simulink library "UR3_Lib"  (R2017a)
settings: Solver=VariableStepAuto  StartTime=0.0  StopTime=10.0  RelTol=1e-3
settings Model: Creator=dscat  LastModifiedBy=dscat

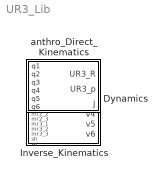
== system UR3_Lib ==
  Dynamics : MATLAB Function  TreatAsAtomicUnit=on
  Inverse_Kinematics : MATLAB Function  TreatAsAtomicUnit=on
  anthro_Direct_Kinematics : MATLAB Function  TreatAsAtomicUnit=on

== matlab function UR3_Lib/Inverse_Kinematics ==
  data: el input; v1 output; mp1 input; mp2 input; mp3 input; mr1_1 input; mr1_2 input; mr1_3 input; mr2_1 input; mr2_2 input; mr2_3 input; mr3_1 input; mr3_2 input; mr3_3 input; sh input; wr input; v2 output; v3 output; v4 output; v5 output; v6 output
function [v1,v2,v3,v4,v5,v6] = Inverse_Kinematics(el,mp1,mp2,mp3,mr1_1,mr1_2,mr1_3,mr2_1,mr2_2,mr2_3,mr3_1,mr3_2,mr3_3,sh,wr)
%#codegen

%    This function was generated by the Symbolic Math Toolbox version 7.2.
%    02-Jun-2018 14:50:33

t6 = mr1_3.*(4.1e1./5.0e2);
t2 = mp1-t6;
t9 = mr2_3.*(4.1e1./5.0e2);
t3 = mp2-t9;
t4 = pi.*(1.0./2.0);
t5 = mp2.*1i;
t7 = mr2_3.*-8.2e-2i;
t8 = t2.^2;
t10 = t3.^2;
t11 = t8+t10;
t12 = 1.0./sqrt(t11);
t13 = t12.*(1.1e1./1.0e2);
t14 = acos(t13);
t15 = sh.*t14;
v1 = t4+t15+angle(mp1-mr1_3.*(4.1e1./5.0e2)+t5+t7);
if nargout > 1
    t16 = mp1+t5-t6+t7;
    t17 = angle(t16);
    t18 = t4+t15+t17;
    t19 = cos(t18);
    t20 = sin(t18);
    t21 = t19.^2;
    t22 = t20.^2;
    t23 = t21+t22;
    t24 = 1.0./t23;
    t25 = mp1.*t20.*(5.0e2./4.1e1);
    t31 = mp2.*t19.*(5.0e2./4.1e1);
    t26 = t25-t31-5.5e1./4.1e1;
    t27 = acos(t26);
    t28 = t27.*wr;
    t29 = sin(t28);
    t30 = 1.0./t29;
    t32 = cos(t28);
    t33 = mr1_2.*t20;
    t38 = mr2_2.*t19;
    t34 = t33-t38;
    t35 = mr1_1.*t20;
    t37 = mr2_1.*t19;
    t36 = t35-t37;
    t44 = t30.*t34;
    t39 = real(-t44);
    t42 = t30.*t36;
    t40 = imag(-t42);
    t41 = t39-t40;
    t116 = t30.*(t33-t38).*-1i;
    t43 = -t116;
    t45 = -t42+t43;
    t46 = abs(t45);
    t47 = t32.^2;
    t48 = real(-t42);
    t49 = imag(-t44);
    t50 = t48+t49;
    t51 = 1.0./t46.^2;
    t52 = t29.^2;
    t53 = t50.^2;
    t54 = t41.^2;
    t55 = 1.0./t46;
    t56 = t47.*t51.*t53;
    t57 = t51.*t52.*t53;
    t58 = t47.*t51.*t54;
    t59 = t51.*t52.*t54;
    t60 = t56+t57+t58+t59;
    t61 = 1.0./t60;
    t63 = t47.*t50.*t55.*8.3e1;
    t64 = t29.*t41.*t55.*1.1e2;
    t65 = t50.*t52.*t55.*8.3e1;
    t66 = t63-t64+t65;
    t67 = t29.*t50.*t55.*1.1e2;
    t68 = t47+t52;
    t69 = 1.0./t68;
    t70 = t32.*5.5e1;
    t71 = t47.*4.1e1;
    t72 = t52.*4.1e1;
    t73 = t70+t71+t72;
    t81 = mr1_1.*t19.*t24;
    t82 = mr2_1.*t20.*t24;
    t83 = t81+t82;
    t84 = mp1.*t19.*t24;
    t85 = mp2.*t20.*t24;
    t86 = mr1_3.*t19.*t24;
    t87 = mr2_3.*t20.*t24;
    t88 = t86+t87;
    t89 = t69.*t73.*t88.*(1.0./5.0e2);
    t90 = mr1_2.*t19.*t24;
    t91 = mr2_2.*t20.*t24;
    t92 = t90+t91;
    t93 = t61.*t66.*t92.*(1.0./1.0e3);
    t62 = t84+t85-t89-t93+t61.*t83.*(t67+(t41.*t52.*8.3e1)./abs(t43-t30.*t36)+(t41.*t47.*8.3e1)./abs(t30.*t34.*1i-t30.*t36)).*(1.0./1.0e3);
    t75 = mr3_2.*t61.*t66.*(1.0./1.0e3);
    t76 = t41.*t47.*t55.*8.3e1;
    t77 = t41.*t52.*t55.*8.3e1;
    t78 = t67+t76+t77;
    t79 = mr3_1.*t61.*t78.*(1.0./1.0e3);
    t80 = mr3_3.*t69.*t73.*(1.0./5.0e2);
    t74 = mp3-t75+t79-t80;
    t97 = t61.*t78.*t83.*(1.0./1.0e3);
    t94 = t84+t85-t89-t93+t97;
    t95 = t74.^2;
    t98 = t94.^2;
    t100 = t98.*9.620564919572077;
    t101 = t95.*9.620564919572077;
    t96 = t100+t101-1.009245362887709;
    t99 = t95.*(1.25e2./6.1e1);
    t102 = t96.^2;
    t103 = -t102+1.0;
    t104 = sqrt(t103);
    t105 = t95+t98;
    t106 = 1.0./t105;
    t107 = el.*t104.*1i;
    t108 = t100+t101+t107-1.009245362887709;
    t109 = angle(t108);
    t110 = t98.*(1.25e2./6.1e1);
    t111 = t99+t110+2.903073770491803e-2;
    t112 = t94.*t111;
    t113 = el.*t74.*t104.*(2.13e2./1.0e3);
    t114 = t112+t113;
    t115 = t106.*t114.*1i;
    v2 = -angle(t115+t106.*(t74.*(t99+t62.^2.*(1.25e2./6.1e1)+2.903073770491803e-2)-el.*t94.*t104.*(2.13e2./1.0e3)));
end
if nargout > 2
    v3 = t109;
end
if nargout > 3
    v4 = -t109+angle(t115+t106.*(t74.*t111-el.*t94.*t104.*(2.13e2./1.0e3)))+angle(-mr3_1.*t41.*t55+mr3_2.*t50.*t55+mr1_1.*t19.*t41.*t55.*1i-mr1_2.*t19.*t50.*t55.*1i+mr2_1.*t20.*t41.*t55.*1i-mr2_2.*t20.*t50.*t55.*1i);
end
if nargout > 4
    v5 = t28;
end
if nargout > 5
    v6 = angle(t116+t30.*(t35-t37));
end

== matlab function UR3_Lib/anthro_Direct_Kinematics ==
  data: q1 input; UR3_R output; q2 input; q3 input; q4 input; q5 input; q6 input; UR3_p output; J output
function [UR3_R,UR3_p,J] = anthro_Direct_Kinematics(q1,q2,q3,q4,q5,q6)
%#codegen

%    This function was generated by the Symbolic Math Toolbox version 7.2.
%    02-Jun-2018 14:45:26

t2 = cos(q1);
t3 = cos(q2);
t4 = cos(q5);
t5 = cos(q3);
t6 = sin(q4);
t7 = cos(q4);
t8 = sin(q2);
t9 = sin(q3);
t10 = sin(q6);
t11 = sin(q1);
t12 = sin(q5);
t13 = t11.*t12;
t14 = t2.*t3.*t4.*t6.*t9;
t15 = t2.*t4.*t5.*t6.*t8;
t16 = t2.*t4.*t7.*t8.*t9;
t17 = t13+t14+t15+t16-t2.*t3.*t4.*t5.*t7;
t18 = q2+q3+q4;
t19 = sin(t18);
t20 = cos(q6);
t21 = t3.*t4.*t6.*t9.*t11;
t22 = t4.*t5.*t6.*t8.*t11;
t23 = t4.*t7.*t8.*t9.*t11;
t24 = t21+t22+t23-t2.*t12-t3.*t4.*t5.*t7.*t11;
t25 = q2+q3+q4+q6;
t26 = q2+q3+q4-q6;
t27 = q2+q3+q4+q5;
t28 = cos(t27);
t29 = q2+q3+q4-q5;
t30 = cos(t29);
t31 = t6.*t8.*t9.*t11.*(8.3e1./1.0e3);
t32 = t3.*t5.*t7.*t11.*t12.*(4.1e1./5.0e2);
t33 = cos(t18);
t34 = t33.*(8.3e1./1.0e3);
t35 = q2+q3;
t36 = cos(t35);
t37 = t36.*(2.13e2./1.0e3);
t38 = t3.*(6.1e1./2.5e2);
t39 = t30.*(4.1e1./1.0e3);
t41 = t28.*(4.1e1./1.0e3);
t40 = t34+t37+t38+t39-t41;
t42 = t2.*t4.*(4.1e1./5.0e2);
t43 = t3.*t5.*t6.*t11.*(8.3e1./1.0e3);
t44 = t3.*t7.*t9.*t11.*(8.3e1./1.0e3);
t45 = t5.*t7.*t8.*t11.*(8.3e1./1.0e3);
t46 = t3.*t6.*t9.*t11.*t12.*(4.1e1./5.0e2);
t47 = t5.*t6.*t8.*t11.*t12.*(4.1e1./5.0e2);
t48 = t7.*t8.*t9.*t11.*t12.*(4.1e1./5.0e2);
t49 = t34+t39-t41;
t50 = t3.*t5.*t7.*t11.*t12;
t51 = t30.*(1.0./2.0);
t52 = t11.*(1.1e1./1.0e2);
t53 = t4.*t11.*(4.1e1./5.0e2);
t54 = t2.*t6.*t8.*t9.*(8.3e1./1.0e3);
t55 = t2.*t3.*t5.*t7.*t12.*(4.1e1./5.0e2);
t60 = t2.*t3.*t5.*t6.*(8.3e1./1.0e3);
t61 = t2.*t3.*t7.*t9.*(8.3e1./1.0e3);
t62 = t2.*t5.*t7.*t8.*(8.3e1./1.0e3);
t63 = t2.*t3.*t6.*t9.*t12.*(4.1e1./5.0e2);
t64 = t2.*t5.*t6.*t8.*t12.*(4.1e1./5.0e2);
t65 = t2.*t7.*t8.*t9.*t12.*(4.1e1./5.0e2);
t75 = t2.*t8.*(6.1e1./2.5e2);
t76 = t2.*t3.*t9.*(2.13e2./1.0e3);
t77 = t2.*t5.*t8.*(2.13e2./1.0e3);
t56 = t52+t53+t54+t55-t60-t61-t62-t63-t64-t65-t75-t76-t77;
t57 = t34+t37+t39-t41;
t58 = q1+q2+q3+q4;
t59 = -q1+q2+q3+q4;
t66 = t4.*t11;
t67 = t2.*t3.*t5.*t7.*t12;
UR3_R = reshape([t17.*t20+t2.*t10.*t19,t20.*t24+t10.*t11.*t19,sin(t25).*(-1.0./2.0)+sin(t26).*(1.0./2.0)-t4.*t19.*t20,-t10.*t17+t2.*t19.*t20,-t10.*t24+t11.*t19.*t20,cos(t25).*(-1.0./2.0)-cos(t26).*(1.0./2.0)+t4.*t10.*t19,t66+t67-t2.*t3.*t6.*t9.*t12-t2.*t5.*t6.*t8.*t12-t2.*t7.*t8.*t9.*t12,t50-t2.*t4-t3.*t6.*t9.*t11.*t12-t5.*t6.*t8.*t11.*t12-t7.*t8.*t9.*t11.*t12,t28.*(-1.0./2.0)+t51],[3,3]);
if nargout > 1
    UR3_p = [t56;t2.*(-1.1e1./1.0e2)+t31+t32-t2.*t4.*(4.1e1./5.0e2)-t8.*t11.*(6.1e1./2.5e2)-t3.*t9.*t11.*(2.13e2./1.0e3)-t5.*t8.*t11.*(2.13e2./1.0e3)-t3.*t5.*t6.*t11.*(8.3e1./1.0e3)-t3.*t7.*t9.*t11.*(8.3e1./1.0e3)-t5.*t7.*t8.*t11.*(8.3e1./1.0e3)-t3.*t6.*t9.*t11.*t12.*(4.1e1./5.0e2)-t5.*t6.*t8.*t11.*t12.*(4.1e1./5.0e2)-t7.*t8.*t9.*t11.*t12.*(4.1e1./5.0e2);t40];
end
if nargout > 2
    t68 = t28.*(1.0./2.0);
    t69 = t51-t68;
    t70 = t2.*(1.1e1./1.0e2);
    t71 = t8.*t11.*(6.1e1./2.5e2);
    t72 = t3.*t9.*t11.*(2.13e2./1.0e3);
    t73 = t5.*t8.*t11.*(2.13e2./1.0e3);
    t74 = -t31-t32+t42+t43+t44+t45+t46+t47+t48+t70+t71+t72+t73;
    t78 = sin(t35);
    t79 = t78.*2.13e2;
    t80 = t8.*2.44e2;
    t81 = t79+t80;
    t82 = cos(t58);
    t83 = t82.*(1.0./2.0);
    t84 = cos(t59);
    t104 = t84.*(1.0./2.0);
    t85 = t83-t104;
    t86 = -t53-t54-t55+t60+t61+t62+t63+t64+t65;
    t87 = sin(t58);
    t88 = t87.*(1.0./2.0);
    t89 = sin(t59);
    t90 = t89.*(1.0./2.0);
    t91 = t88+t90;
    t92 = -t31-t32+t42+t43+t44+t45+t46+t47+t48;
    t93 = -t53-t55+t63+t64+t65;
    t94 = t2.*t4;
    t95 = t3.*t6.*t9.*t11.*t12;
    t96 = t5.*t6.*t8.*t11.*t12;
    t97 = t7.*t8.*t9.*t11.*t12;
    t98 = -t50+t94+t95+t96+t97;
    t99 = t2.*t3.*t6.*t9.*t12;
    t100 = t2.*t5.*t6.*t8.*t12;
    t101 = t2.*t7.*t8.*t9.*t12;
    t102 = -t66-t67+t99+t100+t101;
    t103 = -t32+t42+t46+t47+t48;
    J = reshape([t74,t56,0.0,0.0,0.0,1.0,-t2.*t40,-t11.*t40,-t11.*t74-t2.*(-t52-t53-t54-t55+t60+t61+t62+t63+t64+t65+t75+t76+t77),t11,-t2,0.0,-t2.*t57,-t11.*t57,-t2.*(-t52-t53-t54-t55+t60+t61+t62+t63+t64+t65+t76+t77)-t11.*(-t31-t32+t42+t43+t44+t45+t46+t47+t48+t70+t72+t73),t11,-t2,0.0,-t2.*t49,-t11.*t49,-t11.*(-t31-t32+t42+t43+t44+t45+t46+t47+t48+t70+t71+t72+t73-t11.*t81.*(1.0./1.0e3))-t2.*(-t52-t53-t54-t55+t60+t61+t62+t63+t64+t65+t75+t76+t77-t2.*t81.*(1.0./1.0e3)),t11,-t2,0.0,t33.*t92+t49.*t85,-t33.*t86+t49.*t91,t85.*t86+t91.*t92,-t88-t90,t85,t33,t69.*t103-t98.*(t39-t41),-t69.*t93+t102.*(t39-t41),-t93.*t98+t102.*t103,t66+t67-t99-t100-t101,t50-t94-t95-t96-t97,t69],[6,6]);
end

== matlab function UR3_Lib/Dynamics ==
  data: dq1 input; G output; dq2 input; dq3 input; dq4 input; dq5 input; dq6 input; q2 input; q3 input; q4 input; q5 input; q6 input; C_dq output; B output
function [G,C_dq,B] = Dynamics(dq1,dq2,dq3,dq4,dq5,dq6,q2,q3,q4,q5,q6)
%#codegen

%    This function was generated by the Symbolic Math Toolbox version 7.2.
%    02-Jun-2018 15:14:17

t2 = cos(q2);
t3 = sin(q3);
t4 = cos(q3);
t5 = sin(q2);
t6 = sin(q4);
t7 = cos(q5);
t8 = cos(q4);
t9 = t2.*t3.*(9.81e2./1.0e2);
t10 = t4.*t5.*(9.81e2./1.0e2);
t11 = t9+t10;
t12 = t8.*t11;
t13 = t2.*t4.*(9.81e2./1.0e2);
t17 = t3.*t5.*(9.81e2./1.0e2);
t14 = t13-t17;
t15 = t6.*t14;
t16 = t12+t15;
t18 = cos(q6);
t19 = sin(q6);
t20 = t6.*t11;
t22 = t8.*t14;
t21 = t20-t22;
t23 = sin(q5);
t24 = t7.*t16.*3.3852e-1;
t25 = t19.*t21.*1.6113e-1;
t31 = t7.*t16.*t18.*1.6113e-1;
t26 = t25-t31;
t27 = t18.*t21.*1.6113e-1;
t28 = t7.*t16.*t19.*1.6113e-1;
t37 = t27+t28;
t29 = t19.*t37;
t38 = t18.*t26;
t30 = t24+t29-t38;
t32 = t18.*t21.*1.06974207e-2;
t33 = t7.*t16.*t19.*1.06974207e-2;
t34 = t32+t33;
t35 = t19.*t21.*1.06974207e-2;
t40 = t7.*t16.*t18.*1.06974207e-2;
t36 = t35-t40;
t39 = t7.*t16.*4.5395532e-3;
t41 = t23.^2;
t42 = t16.*t41.*5.49615e-2;
t43 = t8.*t11.*3.7397712e-2;
t44 = t6.*t14.*3.7397712e-2;
t45 = t7.*t16.*3.00842724e-2;
t46 = t16.*t23.*4.34580624e-2;
t47 = t18.*t34;
t48 = t19.*t36;
t49 = t6.*t11.*4.5395532e-3;
t63 = t8.*t14.*4.5395532e-3;
t50 = t46+t47+t48+t49-t63;
t51 = t7.*t50;
t52 = t18.*t37.*(1.1e1./1.0e2);
t53 = t6.*t11.*7.4634912e-2;
t54 = t19.*t26.*(1.1e1./1.0e2);
t55 = t2.*t4.*1.02069867636e-1;
t56 = t19.*(t27+t28);
t57 = t24-t38+t56;
t58 = t7.*t57.*(1.1e1./1.0e2);
t59 = t19.*(t32+t33);
t72 = t18.*t36;
t60 = t39+t42+t43+t44+t58+t59-t72;
t61 = t19.*(t27+t28).*(8.3e1./1.0e3);
t76 = t18.*t26.*(8.3e1./1.0e3);
t62 = t45+t61-t76;
t77 = t23.*t62;
t78 = t8.*t14.*7.4634912e-2;
t64 = t51+t52+t53+t54-t77-t78;
t65 = t4.^2;
t66 = t65.*(2.13e2./1.0e3);
t67 = t3.^2;
t68 = t67.*(2.13e2./1.0e3);
t69 = t66+t68-1.1812e-1;
t70 = t23.*t57;
t107 = t7.*t16.*t23.*4.9965e-1;
t71 = t70-t107;
t73 = t8.*t60;
t74 = t2.*t3.*1.02069867636e-1;
t75 = t4.*t5.*1.02069867636e-1;
t79 = t6.*t64;
t80 = t73+t74+t75+t79;
t81 = t7.*t57;
t82 = t16.*t41.*4.9965e-1;
t83 = t8.*t11.*3.2195e-1;
t84 = t6.*t14.*3.2195e-1;
t85 = t81+t82+t83+t84;
t86 = t18.*t37;
t87 = t6.*t11.*6.6047e-1;
t88 = t19.*t26;
t98 = t8.*t14.*6.6047e-1;
t89 = t86+t87+t88-t98;
t90 = t2.^2;
t91 = t90.*(6.1e1./2.5e2);
t92 = t5.^2;
t93 = t92.*(6.1e1./2.5e2);
t94 = t91+t93-1.6e1./1.25e2;
t95 = t2.*t3.*1.03205124e1;
t96 = t4.*t5.*1.03205124e1;
t97 = t8.*t85;
t99 = t6.*t89;
t100 = t95+t96+t97+t99;
t101 = t2.*t4.*1.03205124e1;
t102 = t6.*t85;
t549 = t3.*t5.*1.03205124e1;
t550 = t8.*t89;
t103 = t101+t102-t549-t550;
t104 = t5.*1.165770980163;
t105 = t6.*t60;
t106 = t23.*t57.*1.1812e-1;
t108 = t69.*t71;
t445 = t3.*t5.*1.02069867636e-1;
t446 = t8.*t64;
t447 = t7.*t16.*t23.*5.9018658e-2;
t109 = t55+t105+t106+t108-t445-t446-t447;
t110 = t4.*t80;
t111 = t2.*1.165770980163;
t112 = dq1.*t2.*t3;
t113 = dq1.*t4.*t5;
t114 = t112+t113;
t115 = dq1.*t2.*t4;
t117 = dq1.*t3.*t5;
t116 = t115-t117;
t118 = t8.*t114;
t119 = t6.*t116;
t120 = t118+t119;
t121 = dq1.*dq2.*t2;
t122 = dq1.*dq3.*t2;
t123 = t121+t122;
t124 = dq1.*dq2.*t5;
t125 = dq1.*dq3.*t5;
t126 = t124+t125;
t127 = t8.*t114.*(1.1e1./1.0e2);
t128 = t6.*t116.*(1.1e1./1.0e2);
t129 = t127+t128;
t130 = t6.*t114;
t131 = t6.*t114.*(1.1e1./1.0e2);
t137 = t8.*t116;
t132 = t130-t137;
t164 = t8.*t116.*(1.1e1./1.0e2);
t133 = t131-t164;
t134 = t4.*t123;
t135 = t66+t68;
t136 = dq2+dq3+dq4;
t138 = dq5-t130+t137;
t139 = dq4.*t116;
t172 = t3.*t126;
t140 = t134+t139-t172;
t141 = dq1.^2;
t142 = t91+t93;
t143 = t5.*(9.81e2./1.0e2);
t144 = t2.*t5.*t141.*t142;
t145 = t143+t144;
t146 = dq2+dq3;
t147 = dq2.^2;
t148 = t142.*t147;
t149 = t92.*t141.*t142;
t156 = t2.*(9.81e2./1.0e2);
t150 = t148+t149-t156;
t151 = dq4.*t114;
t152 = t3.*t123;
t153 = t4.*t126;
t154 = t151+t152+t153;
t155 = t4.*t145;
t157 = t114.*t116.*t135;
t181 = t3.*t150;
t158 = t155+t157-t181;
t159 = t7.*t136;
t160 = t23.*t120;
t161 = t159+t160;
t162 = t7.*t120.*(8.3e1./1.0e3);
t179 = t23.*t136.*(8.3e1./1.0e3);
t163 = t162-t179;
t165 = t3.*t145;
t166 = t146.^2;
t167 = t135.*t166;
t168 = t4.*t150;
t169 = t114.^2;
t170 = t135.*t169;
t171 = t165+t167+t168+t170;
t173 = t7.*t120;
t175 = t23.*t136;
t174 = t173-t175;
t176 = dq6+t159+t160;
t177 = t116.*t135.*t146;
t178 = dq1.*dq2.*t2.*t142.*2.0;
t180 = t6.*t140.*(1.1e1./1.0e2);
t182 = t6.*t171;
t183 = t8.*t154.*(1.1e1./1.0e2);
t210 = t8.*t158;
t211 = t129.*t136;
t184 = t180+t182+t183-t210-t211;
t185 = t6.*t154;
t186 = dq5.*t136;
t202 = t8.*t140;
t187 = t185+t186-t202;
t188 = t6.*t158;
t189 = t7.*t136.*(8.3e1./1.0e3);
t190 = t23.*t120.*(8.3e1./1.0e3);
t191 = t189+t190;
t192 = t161.*t191;
t193 = t163.*t174;
t194 = t136.*(t131-t164);
t195 = t8.*t171;
t196 = t8.*t140.*(1.1e1./1.0e2);
t221 = t6.*t154.*(1.1e1./1.0e2);
t197 = t188+t192+t193+t194+t195+t196-t221;
t198 = t6.*t140;
t199 = dq6.*t174;
t200 = t8.*t154;
t201 = t198+t199+t200;
t203 = t7.*t187;
t204 = dq5.*t23.*t120;
t231 = dq6.*t138;
t205 = t203+t204-t231;
t206 = t134-t172;
t207 = t135.*t206;
t215 = t120.*t129;
t216 = t132.*t133;
t208 = t177+t178+t207-t215-t216;
t209 = t23.*t208;
t212 = t7.*t184;
t213 = dq5.*t7.*t120.*(8.3e1./1.0e3);
t232 = t138.*t163;
t233 = t23.*t187.*(8.3e1./1.0e3);
t214 = t209+t212+t213-t232-t233;
t217 = t7.*t120.*1.341e-2;
t264 = t23.*t136.*1.341e-2;
t218 = t217-t264;
t219 = t7.*t120.*5.87e-3;
t245 = t23.*t136.*5.87e-3;
t220 = t219-t245;
t222 = t19.*t197.*1.6113e-1;
t223 = t18.*t201.*1.06974207e-2;
t224 = t18.*t174.*(4.1e1./5.0e2);
t225 = t19.*t138.*(4.1e1./5.0e2);
t226 = t224+t225;
t227 = t18.*t174.*1.561e-2;
t228 = t19.*t138.*1.561e-2;
t229 = t227+t228;
t230 = t176.*t229.*1.6113e-1;
t234 = t18.*t214.*1.6113e-1;
t284 = t176.*t226.*1.6113e-1;
t285 = t19.*t205.*1.06974207e-2;
t235 = t222+t223+t230+t234-t284-t285;
t236 = t19.*t201.*1.06974207e-2;
t237 = t18.*t205.*1.06974207e-2;
t238 = t18.*t138.*(4.1e1./5.0e2);
t270 = t19.*t174.*(4.1e1./5.0e2);
t239 = t238-t270;
t240 = t176.*t239.*1.6113e-1;
t241 = t18.*t138.*1.561e-2;
t272 = t19.*t174.*1.561e-2;
t242 = t241-t272;
t243 = t19.*t214.*1.6113e-1;
t282 = t18.*t197.*1.6113e-1;
t283 = t176.*t242.*1.6113e-1;
t244 = t236+t237+t240+t243-t282-t283;
t246 = t8.*t114.*6.16e-3;
t247 = t6.*t116.*6.16e-3;
t248 = t246+t247;
t249 = dq2.*9.98e-3;
t250 = dq3.*9.98e-3;
t251 = dq4.*9.98e-3;
t252 = t6.*t114.*6.16e-3;
t340 = t8.*t116.*6.16e-3;
t253 = t249+t250+t251+t252-t340;
t254 = t6.*t114.*3.127e-4;
t255 = t7.*t136.*2.67e-5;
t256 = t23.*t120.*2.67e-5;
t347 = dq5.*3.127e-4;
t348 = t8.*t116.*3.127e-4;
t257 = t254+t255+t256-t347-t348;
t258 = t6.*t114.*1.341e-2;
t259 = t7.*t136.*5.87e-3;
t260 = t23.*t120.*5.87e-3;
t262 = dq5.*1.341e-2;
t263 = t8.*t116.*1.341e-2;
t261 = t258+t259+t260-t262-t263;
t265 = t18.*t174;
t266 = t19.*t138;
t267 = t265+t266;
t268 = t18.*t138;
t271 = t19.*t174;
t269 = t268-t271;
t273 = t18.*t138.*5.678e-5;
t312 = t19.*t174.*5.678e-5;
t274 = t273-t312;
t275 = dq6.*8.652000000000001e-5;
t276 = t7.*t136.*8.652000000000001e-5;
t277 = t23.*t120.*8.652000000000001e-5;
t278 = t275+t276+t277;
t279 = t18.*t174.*5.678e-5;
t280 = t19.*t138.*5.678e-5;
t281 = t279+t280;
t286 = t6.*t114.*2.67e-5;
t287 = t7.*t136.*2.449e-4;
t288 = t23.*t120.*2.449e-4;
t381 = dq5.*2.67e-5;
t382 = t8.*t116.*2.67e-5;
t289 = t286+t287+t288-t381-t382;
t290 = t6.*t140.*4.5395532e-3;
t291 = t7.*t184.*3.3852e-1;
t292 = t18.*t235;
t293 = t19.*t244;
t294 = t8.*t154.*4.5395532e-3;
t295 = dq5.*t7.*t120.*3.00842724e-2;
t296 = t8.*t114.*9.98e-3;
t297 = t6.*t116.*9.98e-3;
t298 = t296+t297;
t299 = t7.*t120.*3.462e-4;
t351 = t23.*t136.*3.462e-4;
t300 = t299-t351;
t301 = dq2.*2.61e-4;
t302 = dq3.*2.61e-4;
t303 = dq4.*2.61e-4;
t304 = t6.*t114.*1.99e-5;
t368 = t8.*t116.*1.99e-5;
t305 = t301+t302+t303+t304-t368;
t306 = t267.*t278;
t307 = t19.*t197.*1.06974207e-2;
t308 = t18.*t201.*7.66981760273e-4;
t309 = t176.*t229.*1.06974207e-2;
t310 = t18.*t214.*1.06974207e-2;
t395 = t176.*t281;
t396 = t176.*t226.*1.06974207e-2;
t397 = t19.*t205.*7.66981760273e-4;
t311 = t306+t307+t308+t309+t310-t395-t396-t397;
t313 = t176.*t274;
t314 = t19.*t201.*7.66981760273e-4;
t315 = t18.*t205.*7.66981760273e-4;
t316 = t176.*t239.*1.06974207e-2;
t317 = t19.*t214.*1.06974207e-2;
t392 = t269.*t278;
t393 = t18.*t197.*1.06974207e-2;
t394 = t176.*t242.*1.06974207e-2;
t318 = t313+t314+t315+t316+t317-t392-t393-t394;
t319 = dq1.*t2.*t3.*9.89e-3;
t320 = dq1.*t4.*t5.*9.89e-3;
t321 = t319+t320;
t322 = t174.*t218.*3.3852e-1;
t323 = t226.*t267.*1.6113e-1;
t324 = t239.*t269.*1.6113e-1;
t325 = t23.*t184.*4.9965e-1;
t326 = t7.*t187.*4.34580624e-2;
t327 = dq5.*t23.*t120.*4.34580624e-2;
t331 = t7.*t208.*4.9965e-1;
t332 = t138.*t261.*3.3852e-1;
t333 = t138.*t191.*4.9965e-1;
t334 = t229.*t267.*1.6113e-1;
t335 = t242.*t269.*1.6113e-1;
t328 = t322+t323+t324+t325+t326+t327-t331-t332-t333-t334-t335;
t329 = t23.*t208.*3.3852e-1;
t405 = t161.*t218.*3.3852e-1;
t406 = t138.*t163.*3.3852e-1;
t407 = t138.*t220.*3.3852e-1;
t408 = t23.*t187.*3.00842724e-2;
t330 = t290+t291+t292+t293+t294+t295+t329-t405-t406-t407-t408;
t336 = dq2.*1.1812e-1;
t337 = dq3.*1.1812e-1;
t338 = dq1.*t2.*t4.*9.89e-3;
t404 = dq1.*t3.*t5.*9.89e-3;
t339 = t336+t337+t338-t404;
t341 = dq2.*(1.6e1./1.25e2);
t342 = dq1.*t2.*8.721e-2;
t343 = t341+t342;
t344 = dq1.*t2.*t3.*1.1812e-1;
t345 = dq1.*t4.*t5.*1.1812e-1;
t346 = t344+t345;
t349 = t6.*t140.*4.30130092884e-4;
t350 = t23.*t208.*3.00842724e-2;
t352 = t267.*t274;
t353 = t7.*t184.*3.00842724e-2;
t354 = t18.*t235.*(8.3e1./1.0e3);
t355 = t19.*t244.*(8.3e1./1.0e3);
t356 = t8.*t154.*4.30130092884e-4;
t357 = dq5.*t7.*t120.*3.005009288188e-3;
t454 = t174.*t257;
t455 = t161.*t218.*3.00842724e-2;
t456 = t138.*t163.*3.00842724e-2;
t457 = t138.*t220.*3.00842724e-2;
t458 = t138.*t300;
t459 = t269.*t281;
t460 = t23.*t187.*3.005009288188e-3;
t358 = t349+t350+t352+t353+t354+t355+t356+t357-t454-t455-t456-t457-t458-t459-t460;
t359 = t23.*t358;
t360 = t6.*t158.*7.4634912e-2;
t361 = t161.*t261.*3.72372e-2;
t362 = t161.*t191.*3.72372e-2;
t363 = t163.*t174.*3.72372e-2;
t364 = t174.*t220.*3.72372e-2;
t365 = t120.*t298.*3.7397712e-2;
t366 = t8.*t171.*7.4634912e-2;
t367 = t135.*t206.*3.213061e-3;
t369 = t136.*t253.*3.7397712e-2;
t370 = dq2.*1.99e-5;
t371 = dq3.*1.99e-5;
t372 = dq4.*1.99e-5;
t373 = t6.*t114.*2.318e-4;
t467 = t8.*t116.*2.318e-4;
t374 = t370+t371+t372+t373-t467;
t375 = t136.*t374;
t376 = t161.*t257;
t377 = t7.*t208.*4.34580624e-2;
t378 = t6.*t158.*4.5395532e-3;
t379 = t161.*t261.*4.5395532e-3;
t380 = t138.*t261.*3.00842724e-2;
t383 = t138.*t289;
t384 = t161.*t191.*4.5395532e-3;
t385 = t163.*t174.*4.5395532e-3;
t386 = t174.*t220.*4.5395532e-3;
t387 = t138.*t191.*4.34580624e-2;
t388 = t8.*t171.*4.5395532e-3;
t389 = dq6.*t138.*1.68983e-4;
t390 = t229.*t267.*1.337379e-2;
t391 = t242.*t269.*1.337379e-2;
t398 = t19.*t311;
t399 = t8.*t140.*4.99350852e-4;
t400 = t19.*t235.*(1.1e1./1.0e2);
t401 = t8.*t140.*8.7660765747e-3;
t402 = t116.*t135.*t146.*3.213061e-3;
t403 = dq1.*dq2.*t2.*t142.*6.426122e-3;
t409 = dq2.*8.3e-3;
t410 = dq3.*8.3e-3;
t411 = dq1.*t3.*t5.*4.0e-4;
t480 = dq1.*t2.*t4.*4.0e-4;
t412 = t409+t410+t411-t480;
t413 = t6.*t154.*3.213061e-3;
t414 = t114.*t321.*1.05204;
t415 = t120.*t129.*3.2195e-1;
t416 = t120.*t248.*3.2195e-1;
t417 = t7.*t328;
t418 = t4.*t123.*1.242669648e-1;
t419 = t116.*t339.*1.05204;
t420 = t132.*t253.*3.2195e-1;
t421 = t132.*t133.*3.2195e-1;
t422 = t6.*t140.*4.949493634332e-3;
t423 = t23.*t208.*4.5395532e-3;
t424 = t174.*t289;
t425 = t7.*t330.*(1.1e1./1.0e2);
t426 = t23.*t328.*(1.1e1./1.0e2);
t427 = t6.*t171.*3.7397712e-2;
t428 = dq6.*t174.*1.68983e-4;
t429 = t120.*t305;
t430 = t7.*t184.*4.5395532e-3;
t431 = t8.*t114.*2.938e-4;
t432 = t6.*t116.*2.938e-4;
t433 = t431+t432;
t434 = t18.*t311;
t435 = t19.*t318;
t436 = t8.*t154.*4.949493634332e-3;
t437 = dq5.*t7.*t120.*4.30130092884e-4;
t438 = t133.*t136.*4.5395532e-3;
t468 = t6.*t154.*4.99350852e-4;
t469 = t174.*t218.*3.00842724e-2;
t470 = t226.*t267.*1.337379e-2;
t471 = t239.*t269.*1.337379e-2;
t472 = t23.*t184.*4.34580624e-2;
t473 = t18.*t318;
t474 = t7.*t187.*4.1906892666e-3;
t475 = dq5.*t23.*t120.*4.1906892666e-3;
t439 = t376+t377+t378+t379+t380+t383+t384+t385+t386+t387+t388+t389+t390+t391+t398+t399+t438-t468-t469-t470-t471-t472-t473-t474-t475;
t440 = t7.*t439;
t441 = t133.*t136.*7.4634912e-2;
t453 = t6.*t154.*8.7660765747e-3;
t461 = dq5.*t136.*1.68983e-4;
t462 = t120.*t129.*3.213061e-3;
t463 = t132.*t133.*3.213061e-3;
t464 = t120.*t248.*3.213061e-3;
t465 = t132.*t305;
t466 = t132.*t253.*3.213061e-3;
t476 = t18.*t244.*(1.1e1./1.0e2);
t477 = t7.*t187.*4.99350852e-4;
t478 = dq5.*t23.*t120.*4.99350852e-4;
t442 = t359+t360+t361+t362+t363+t364+t365+t366+t367+t369+t375+t400+t401+t402+t403+t440+t441-t453-t461-t462-t463-t464-t465-t466-t476-t477-t478;
t443 = t132.*t298.*3.7397712e-2;
t481 = t8.*t158.*3.7397712e-2;
t482 = t161.*t218.*4.5395532e-3;
t483 = t138.*t163.*4.5395532e-3;
t484 = t138.*t220.*4.5395532e-3;
t485 = t129.*t136.*3.7397712e-2;
t486 = t136.*t248.*3.7397712e-2;
t487 = t161.*t300;
t488 = t136.*t433;
t489 = t23.*t187.*4.30130092884e-4;
t444 = t422+t423+t424+t425+t426+t427+t428+t429+t430+t434+t435+t436+t437+t443-t481-t482-t483-t484-t485-t486-t487-t488-t489;
t448 = t4.*t109;
t449 = t23.*t57.*(1.6e1./1.25e2);
t450 = t71.*t94;
t451 = dq4.*t114.*1.68983e-4;
t452 = t4.*t145.*1.04046756e-2;
t479 = t6.*t442;
t490 = dq1.*t2.*t3.*8.5e-3;
t491 = dq1.*t4.*t5.*8.5e-3;
t492 = t490+t491;
t493 = t146.*t492;
t494 = t146.*t321.*1.04046756e-2;
t495 = t114.*t116.*t135.*1.04046756e-2;
t496 = t3.*t145.*1.04046756e-2;
t497 = dq2.*4.0e-4;
t498 = dq3.*4.0e-4;
t499 = dq1.*t3.*t5.*1.2e-3;
t559 = dq1.*t2.*t4.*1.2e-3;
t500 = t497+t498+t499-t559;
t501 = t146.*t500;
t502 = t23.*t330.*1.1812e-1;
t503 = t135.*t166.*1.04046756e-2;
t504 = t4.*t150.*1.04046756e-2;
t505 = t4.*t123.*8.602902241684e-3;
t506 = t116.*t412;
t507 = t135.*t206.*3.8028734e-2;
t508 = t135.*t169.*1.04046756e-2;
t509 = t413+t414+t415+t416+t417+t418+t419+t420+t421-t3.*t126.*1.242669648e-1-t8.*t140.*3.213061e-3-t135.*t206.*1.37399-t23.*t330-t116.*t135.*t146.*1.37399-dq1.*dq2.*t2.*t142.*2.74798;
t510 = t298.*(t130-t137).*3.7397712e-2;
t511 = t422+t423+t424+t425+t426+t427+t428+t429+t430+t434+t435+t436+t437-t481-t482-t483-t484-t485-t486-t487-t488-t489+t510;
t512 = t8.*t140.*3.7952676532e-4;
t513 = t116.*t135.*t146.*3.8028734e-2;
t514 = dq1.*dq2.*t2.*t142.*7.6057468e-2;
t515 = dq2.*(3.0./2.0e2);
t516 = dq1.*t2.*3.0e-4;
t517 = t515+t516;
t518 = t5.*1.33674003e1;
t519 = t6.*t140.*3.7397712e-2;
t520 = t7.*t330;
t521 = t23.*t328;
t522 = t6.*t171.*3.2195e-1;
t523 = t8.*t154.*3.7397712e-2;
t524 = t6.*t158.*6.6047e-1;
t525 = t161.*t261.*3.3852e-1;
t526 = t161.*t191.*3.3852e-1;
t527 = t163.*t174.*3.3852e-1;
t528 = t174.*t220.*3.3852e-1;
t529 = t120.*t298.*3.2195e-1;
t530 = t8.*t171.*6.6047e-1;
t531 = t136.*t253.*3.2195e-1;
t532 = t19.*t235;
t533 = t8.*t140.*7.4634912e-2;
t534 = t132.*t298.*3.2195e-1;
t542 = t8.*t158.*3.2195e-1;
t543 = t129.*t136.*3.2195e-1;
t544 = t136.*t248.*3.2195e-1;
t535 = t519+t520+t521+t522+t523+t534-t542-t543-t544;
t536 = t133.*t136.*6.6047e-1;
t545 = t6.*t154.*7.4634912e-2;
t546 = t18.*t244;
t547 = t7.*t187.*4.5395532e-3;
t548 = dq5.*t23.*t120.*4.5395532e-3;
t537 = t524+t525+t526+t527+t528+t529+t530+t531+t532+t533+t536-t545-t546-t547-t548;
t538 = t116.*t346.*1.05204;
t539 = t3.*t150.*1.05204;
t540 = t3.*t123.*1.04046756e-2;
t541 = t4.*t126.*1.04046756e-2;
t551 = t3.*t145.*1.05204;
t552 = t135.*t166.*1.05204;
t553 = t4.*t150.*1.05204;
t554 = t4.*t123.*1.04046756e-2;
t555 = t135.*t169.*1.05204;
t556 = t298.*(t130-t137).*3.2195e-1;
t557 = t519+t520+t521+t522+t523-t542-t543-t544+t556;
t558 = t8.*t537;
t560 = t6.*(t86+t87+t88-t98);
t561 = t95+t96+t97+t560;
t562 = t8.*t557;
t582 = t4.*t145.*1.05204;
t583 = t6.*t537;
t584 = t146.*t321.*1.05204;
t585 = t114.*t116.*t135.*1.05204;
t563 = t538+t539+t540+t541+t562-t582-t583-t584-t585;
t564 = t136.*(t131-t164).*4.5395532e-3;
t565 = t376+t377+t378+t379+t380+t383+t384+t385+t386+t387+t388+t389+t390+t391+t398+t399-t468-t469-t470-t471-t472-t473-t474-t475+t564;
t566 = t3.*t103.*(1.6e1./1.25e2);
t567 = dq2.*3.0e-4;
t568 = dq1.*t2.*2.1e-3;
t569 = t567+t568;
t570 = t7.*t358;
t571 = t7.*t62;
t572 = t6.*t140.*3.9312916576e-4;
t573 = t8.*t85.*1.1812e-1;
t574 = dq5.*t120.*1.68983e-4;
t575 = t298.*(t130-t137).*3.213061e-3;
t576 = t3.*t123.*4.0e-4;
t577 = t69.*t561;
t578 = t6.*t171.*3.213061e-3;
t579 = t4.*t126.*4.0e-4;
t580 = t8.*t557.*1.1812e-1;
t581 = t8.*t11.*3.213061e-3;
t586 = t69.*t563;
t587 = t6.*t14.*3.213061e-3;
t588 = t433.*(t130-t137);
t589 = t23.*(t46+t47+t48+t49-t63);
t590 = t6.*(t86+t87+t88-t98).*1.1812e-1;
t591 = t8.*t154.*3.9312916576e-4;
t592 = t19.*t34;
G = [-t5.*(t111+t448+t449+t450+t3.*t80-t7.*t16.*t23.*6.39552e-2)+t2.*(t104+t110-t3.*(t55+t6.*(t39+t42+t43+t44+t592+t7.*t30.*(1.1e1./1.0e2)-t18.*t36)+t69.*(t23.*t30-t7.*t16.*t23.*4.9965e-1)-t3.*t5.*1.02069867636e-1+t23.*t30.*1.1812e-1-t8.*(t51+t52+t53+t54-t23.*(t45-t18.*t26.*(8.3e1./1.0e3)+t19.*t37.*(8.3e1./1.0e3))-t8.*t14.*7.4634912e-2)-t7.*t16.*t23.*5.9018658e-2)),t566-t94.*(t518+t4.*t100-t3.*t103)-t8.*t11.*3.213061e-3-t6.*t14.*3.213061e-3-t7.*t62-t23.*t50-t8.*t85.*1.1812e-1-t6.*t89.*1.1812e-1-t4.*t100.*(1.6e1./1.25e2)-t69.*t100,t8.*t11.*(-3.213061e-3)-t6.*t14.*3.213061e-3-t7.*t62-t23.*t50-t8.*t85.*1.1812e-1-t6.*t89.*1.1812e-1-t69.*t100,t8.*t11.*(-3.213061e-3)-t6.*t14.*3.213061e-3-t7.*t62-t23.*t50,t39+t59-t72,0.0];
if nargout > 1
    C_dq = [-t5.*(t111+dq2.*t343.*1.188349623e-1+dq2.*t569+t94.*(t413+t414+t415+t416+t417+t418+t419+t420+t421-t3.*t126.*1.242669648e-1-t8.*t140.*3.213061e-3+t92.*t141.*1.188349623e-1-t135.*t206.*1.37399-t23.*t330+dq1.*dq2.*t2.*1.7441664e-1+dq1.*t2.*t343.*1.36263-t116.*t135.*t146.*1.37399-dq1.*dq2.*t2.*t142.*5.47324)+t4.*t123.*1.59061714944e-2-t3.*t126.*1.59061714944e-2-t8.*t140.*4.11271808e-4+t6.*t154.*4.11271808e-4+t92.*t141.*1.52108751744e-2+t120.*t129.*4.12096e-2+t132.*t133.*4.12096e-2-t142.*t147.*1.188349623e-1+t7.*t328.*(1.6e1./1.25e2)-t135.*t206.*1.7587072e-1-t23.*t330.*(1.6e1./1.25e2)+t120.*t248.*4.12096e-2+t132.*t253.*4.12096e-2+t114.*t321.*1.3466112e-1+t116.*t339.*1.3466112e-1-t4.*(t496+t501+t502+t503+t504+t505+t506+t507+t508+t512+t513+t514-dq4.*t116.*1.68983e-4-t3.*t126.*8.602902241684e-3-t6.*t154.*3.7952676532e-4-t120.*t129.*3.8028734e-2-t132.*t133.*3.8028734e-2-t7.*t328.*1.1812e-1-t120.*t248.*3.8028734e-2-t132.*t253.*3.8028734e-2+t6.*t444+t8.*t442-t114.*t346.*1.04046756e-2-t146.*t339.*1.04046756e-2-t69.*t509)+t3.*(t451+t452+t479+t493+t494+t495-t3.*t123.*1.302902241684e-3-t4.*t126.*1.302902241684e-3-t3.*t150.*1.04046756e-2-t8.*t444-t116.*t346.*1.04046756e-2-t114.*t412)-dq1.*dq2.*t2.*2.5663597062183e-2-dq1.*dq3.*t2.*1.68983e-4-dq1.*t2.*t517-t92.*t141.*t142.*1.188349623e-1-t116.*t135.*t146.*1.7587072e-1-dq1.*dq2.*t2.*t142.*3.5174144e-1)-t2.*(t104+t110-t3.*t109)+t2.*(t104+t3.*(t496+t501+t502+t503+t504+t505+t506+t507+t508+t512+t513+t514+t8.*(t359+t360+t361+t362+t363+t364+t365+t366+t367+t369+t375+t400+t401+t402+t403-t453-t461-t462-t463-t464-t465-t466-t476-t477-t478+t7.*t565+t136.*(t131-t164).*7.4634912e-2)-dq4.*t116.*1.68983e-4-t3.*t126.*8.602902241684e-3-t6.*t154.*3.7952676532e-4-t120.*t129.*3.8028734e-2-t132.*t133.*3.8028734e-2-t7.*t328.*1.1812e-1-t120.*t248.*3.8028734e-2-t132.*t253.*3.8028734e-2-t114.*t346.*1.04046756e-2-t146.*t339.*1.04046756e-2+t6.*t511-t69.*t509)+t4.*(t451+t452+t479+t493+t494+t495-t3.*t123.*1.302902241684e-3-t4.*t126.*1.302902241684e-3-t3.*t150.*1.04046756e-2-t116.*t346.*1.04046756e-2-t8.*t511-t114.*t412)+dq1.*dq2.*t5.*1.32e-2-dq1.*dq3.*t5.*1.68983e-4-dq1.*t5.*t517-t2.*t5.*t141.*1.52108751744e-2+t2.*t5.*t141.*t142.*1.188349623e-1)+t5.*(t111+t448+t449+t450+t3.*(t73+t74+t75+t6.*(t51+t52+t53+t54-t77-t78))-t7.*t16.*t23.*6.39552e-2),-t566+t570+t571+t572+t573+t574+t575+t576+t577+t578+t579+t580+t581+t586+t587+t588+t589+t590+t591+t94.*(t518-t3.*t103+t4.*t561)-t8.*t158.*3.213061e-3-t129.*t136.*3.213061e-3-t136.*t248.*3.213061e-3-t120.*t374-t6.*t537.*1.1812e-1+t4.*t561.*(1.6e1./1.25e2)+t4.*t563.*(1.6e1./1.25e2)-t23.*t565-t116.*t492-t114.*t500-t94.*(t518+t3.*(t551+t552+t553+t554+t555+t558-t3.*t126.*1.04046756e-2-t114.*t346.*1.05204-t146.*t339.*1.05204+t6.*t535)-t4.*(t538+t539+t540+t541-t4.*t145.*1.05204-t146.*t321.*1.05204-t6.*t537+t8.*t535-t114.*t116.*t135.*1.05204)-t2.*t5.*t141.*1.7441664e-1+t2.*t5.*t141.*t142.*1.36263)-t3.*(t551+t552+t553+t554+t555+t558-t3.*t126.*1.04046756e-2-t114.*t346.*1.05204-t146.*t339.*1.05204+t6.*t557).*(1.6e1./1.25e2)-dq1.*dq2.*t5.*3.0e-4+dq1.*t5.*t569-t2.*t5.*t141.*1.53e-2,t570+t571+t572+t573+t574+t575+t576+t577+t578+t579+t580+t581+t586+t587+t588+t589+t590+t591-t8.*t158.*3.213061e-3-t129.*t136.*3.213061e-3-t136.*t248.*3.213061e-3-t120.*t374-t6.*t537.*1.1812e-1-t23.*t565-t116.*t492-t114.*t500,t570+t571+t572+t574+t575+t578+t581+t587+t588+t589+t591-t8.*t158.*3.213061e-3-t129.*t136.*3.213061e-3-t136.*t248.*3.213061e-3-t120.*t374-t23.*t565,-t39-t423-t424-t428-t430-t434-t435-t437+t482+t483+t484+t487+t489-t592-t6.*t140.*5.42558408412e-4-t8.*t154.*5.42558408412e-4+t18.*(t35-t40),t352-t459-t23.*t187.*2.55503e-4+dq5.*t7.*t120.*2.55503e-4];
end
if nargout > 2
    t593 = t2.*t4;
    t602 = t3.*t5;
    t594 = t593-t602;
    t595 = t2.*t3;
    t596 = t4.*t5;
    t597 = t595+t596;
    t598 = t135.*t597;
    t599 = t5.*t142;
    t600 = t598+t599;
    t601 = t8.*t597;
    t603 = t6.*t594;
    t604 = t601+t603;
    t605 = t7.*t604.*4.34580624e-2;
    t606 = t8.*t594.*(1.1e1./1.0e2);
    t611 = t6.*t597.*(1.1e1./1.0e2);
    t607 = t606-t611;
    t608 = t23.*t607.*4.9965e-1;
    t609 = t7.*t600.*4.9965e-1;
    t610 = t605+t608+t609;
    t612 = t23.*t600;
    t613 = t23.*t604.*(8.3e1./1.0e3);
    t621 = t7.*t607;
    t614 = t612+t613-t621;
    t615 = t8.*t597.*(1.1e1./1.0e2);
    t616 = t6.*t594.*(1.1e1./1.0e2);
    t617 = t615+t616;
    t618 = t8.*t594;
    t620 = t6.*t597;
    t619 = t618-t620;
    t622 = t18.*t617.*1.06974207e-2;
    t623 = t19.*t619.*7.66981760273e-4;
    t624 = t7.*t18.*t604.*7.66981760273e-4;
    t649 = t19.*t614.*1.06974207e-2;
    t625 = t622+t623+t624-t649;
    t626 = t19.*t617.*1.06974207e-2;
    t627 = t18.*t614.*1.06974207e-2;
    t628 = t7.*t19.*t604.*7.66981760273e-4;
    t651 = t18.*t619.*7.66981760273e-4;
    t629 = t626+t627+t628-t651;
    t630 = t18.*t617.*1.6113e-1;
    t631 = t19.*t619.*1.06974207e-2;
    t632 = t7.*t18.*t604.*1.06974207e-2;
    t639 = t19.*t614.*1.6113e-1;
    t633 = t630+t631+t632-t639;
    t634 = t19.*t617.*1.6113e-1;
    t635 = t18.*t614.*1.6113e-1;
    t636 = t7.*t19.*t604.*1.06974207e-2;
    t638 = t18.*t619.*1.06974207e-2;
    t637 = t634+t635+t636-t638;
    t640 = t23.*t600.*3.3852e-1;
    t641 = t23.*t604.*3.00842724e-2;
    t642 = t18.*t637;
    t643 = t6.*t597.*4.5395532e-3;
    t674 = t7.*t607.*3.3852e-1;
    t675 = t8.*t594.*4.5395532e-3;
    t676 = t19.*t633;
    t644 = t640+t641+t642+t643-t674-t675-t676;
    t645 = t7.*t604.*4.99350852e-4;
    t646 = t135.*t597.*3.213061e-3;
    t647 = t7.*t604.*4.1906892666e-3;
    t648 = t23.*t607.*4.34580624e-2;
    t650 = t18.*t625;
    t652 = t19.*t629;
    t653 = t8.*t597.*4.99350852e-4;
    t654 = t6.*t594.*4.99350852e-4;
    t655 = t7.*t600.*4.34580624e-2;
    t656 = t647+t648+t650+t652+t653+t654+t655;
    t657 = t7.*t656;
    t658 = t18.*t633.*(1.1e1./1.0e2);
    t659 = t8.*t597.*8.7660765747e-3;
    t660 = t19.*t637.*(1.1e1./1.0e2);
    t661 = t23.*t600.*3.00842724e-2;
    t662 = t23.*t604.*3.005009288188e-3;
    t663 = t18.*t637.*(8.3e1./1.0e3);
    t664 = t6.*t597.*4.30130092884e-4;
    t689 = t7.*t607.*3.00842724e-2;
    t690 = t8.*t594.*4.30130092884e-4;
    t691 = t19.*t633.*(8.3e1./1.0e3);
    t665 = t661+t662+t663+t664-t689-t690-t691;
    t666 = t23.*t665;
    t667 = t6.*t594.*8.7660765747e-3;
    t668 = t5.*t142.*3.213061e-3;
    t669 = t645+t646+t657+t658+t659+t660+t666+t667+t668;
    t670 = t23.*t600.*4.5395532e-3;
    t671 = t23.*t604.*4.30130092884e-4;
    t672 = t18.*t629;
    t673 = t6.*t597.*4.949493634332e-3;
    t677 = t7.*t644.*(1.1e1./1.0e2);
    t685 = t23.*t610.*(1.1e1./1.0e2);
    t686 = t7.*t607.*4.5395532e-3;
    t687 = t19.*t625;
    t688 = t8.*t594.*4.949493634332e-3;
    t678 = t670+t671+t672+t673+t677-t685-t686-t687-t688;
    t679 = t7.*t610;
    t680 = t135.*t597.*1.37399;
    t681 = t8.*t597.*3.213061e-3;
    t682 = t6.*t594.*3.213061e-3;
    t683 = t23.*t644;
    t684 = t2.*t4.*1.302902241684e-3;
    t692 = t6.*t669;
    t693 = t684+t692-t3.*t5.*1.302902241684e-3-t8.*t678;
    t694 = t7.*t610.*1.1812e-1;
    t695 = t2.*t3.*8.602902241684e-3;
    t696 = t4.*t5.*8.602902241684e-3;
    t697 = t5.*t142.*1.37399;
    t698 = t679+t680+t681+t682+t683+t697-t2.*t3.*1.242669648e-1-t4.*t5.*1.242669648e-1;
    t699 = t69.*t698;
    t700 = t8.*t669;
    t701 = t6.*t678;
    t702 = t135.*t597.*3.8028734e-2;
    t703 = t8.*t597.*3.7952676532e-4;
    t704 = t6.*t594.*3.7952676532e-4;
    t705 = t5.*t142.*3.8028734e-2;
    t706 = t23.*t644.*1.1812e-1;
    t707 = t694+t695+t696+t699+t700+t701+t702+t703+t704+t705+t706;
    t708 = t4.*t142;
    t709 = t66+t68+t708;
    t710 = t7.*(8.3e1./1.0e3);
    t711 = t8.*t709;
    t718 = t3.*t6.*t142;
    t712 = t711-t718;
    t713 = t7.*t712;
    t714 = t710+t713;
    t715 = t6.*t709;
    t716 = t3.*t8.*t142;
    t717 = t715+t716;
    t719 = t7.*3.00842724e-2;
    t720 = t19.*t23.*1.06974207e-2;
    t721 = t19.*t717.*1.6113e-1;
    t735 = t18.*t714.*1.6113e-1;
    t722 = t720+t721-t735;
    t723 = t18.*t23.*1.06974207e-2;
    t724 = t19.*t714.*1.6113e-1;
    t725 = t18.*t717.*1.6113e-1;
    t726 = t723+t724+t725;
    t727 = t19.*t726;
    t728 = t7.*t712.*3.3852e-1;
    t736 = t18.*t722;
    t729 = t719+t727+t728-t736;
    t730 = t23.*t729;
    t731 = t23.*4.34580624e-2;
    t732 = t23.*t712.*4.9965e-1;
    t733 = t731+t732;
    t770 = t7.*t733;
    t734 = t730-t770;
    t737 = t19.*t23.*7.66981760273e-4;
    t738 = t19.*t717.*1.06974207e-2;
    t746 = t18.*t714.*1.06974207e-2;
    t739 = t737+t738-t746;
    t740 = t18.*t23.*7.66981760273e-4;
    t741 = t19.*t714.*1.06974207e-2;
    t742 = t18.*t717.*1.06974207e-2;
    t743 = t740+t741+t742;
    t744 = t7.*4.30130092884e-4;
    t745 = t23.*t733.*(1.1e1./1.0e2);
    t747 = t19.*t743;
    t748 = t8.*t709.*3.7397712e-2;
    t749 = t7.*t729.*(1.1e1./1.0e2);
    t750 = t7.*t712.*4.5395532e-3;
    t775 = t18.*t739;
    t776 = t3.*t6.*t142.*3.7397712e-2;
    t751 = t744+t745+t747+t748+t749+t750-t775-t776+3.9312916576e-4;
    t752 = t23.*4.99350852e-4;
    t753 = t7.*3.005009288188e-3;
    t754 = t19.*t726.*(8.3e1./1.0e3);
    t755 = t7.*t712.*3.00842724e-2;
    t771 = t18.*t722.*(8.3e1./1.0e3);
    t756 = t753+t754+t755-t771;
    t757 = t23.*4.1906892666e-3;
    t758 = t19.*t739;
    t759 = t6.*t709.*4.5395532e-3;
    t760 = t18.*t743;
    t761 = t23.*t712.*4.34580624e-2;
    t762 = t3.*t8.*t142.*4.5395532e-3;
    t763 = t757+t758+t759+t760+t761+t762;
    t764 = t7.*t763;
    t765 = t6.*t709.*7.4634912e-2;
    t766 = t18.*t726.*(1.1e1./1.0e2);
    t767 = t19.*t722.*(1.1e1./1.0e2);
    t768 = t3.*t8.*t142.*7.4634912e-2;
    t772 = t23.*t756;
    t769 = t752+t764+t765+t766+t767+t768-t772;
    t773 = t8.*t769;
    t774 = t3.*t142.*1.04046756e-2;
    t777 = t7.*t733.*1.1812e-1;
    t778 = t65.*2.2161959028e-3;
    t779 = t67.*2.2161959028e-3;
    t780 = t4.*t142.*1.04046756e-2;
    t781 = t8.*t751;
    t782 = t6.*t769;
    t783 = t778+t779+t780+t781+t782-8.29000281872e-4;
    t784 = t773+t774+t777-t23.*t729.*1.1812e-1-t6.*t751-t69.*t734;
    t785 = t7.*t8.*t135;
    t786 = t710+t785;
    t787 = t6.*t19.*t135.*1.6113e-1;
    t795 = t18.*t786.*1.6113e-1;
    t788 = t720+t787-t795;
    t789 = t19.*t786.*1.6113e-1;
    t790 = t6.*t18.*t135.*1.6113e-1;
    t791 = t723+t789+t790;
    t792 = t19.*t791;
    t793 = t7.*t8.*t135.*3.3852e-1;
    t796 = t18.*t788;
    t794 = t719+t792+t793-t796;
    t797 = t23.*t794;
    t798 = t8.*t23.*t135.*4.9965e-1;
    t799 = t731+t798;
    t827 = t7.*t799;
    t800 = t797-t827;
    t801 = t19.*t786.*1.06974207e-2;
    t802 = t6.*t18.*t135.*1.06974207e-2;
    t803 = t740+t801+t802;
    t804 = t6.*t19.*t135.*1.06974207e-2;
    t807 = t18.*t786.*1.06974207e-2;
    t805 = t737+t804-t807;
    t806 = t7.*t794.*(1.1e1./1.0e2);
    t808 = t19.*t803;
    t809 = t23.*t799.*(1.1e1./1.0e2);
    t810 = t8.*t135.*3.7397712e-2;
    t811 = t7.*t8.*t135.*4.5395532e-3;
    t829 = t18.*t805;
    t812 = t744+t806+t808+t809+t810+t811-t829+3.9312916576e-4;
    t813 = t19.*t791.*(8.3e1./1.0e3);
    t814 = t7.*t8.*t135.*3.00842724e-2;
    t831 = t18.*t788.*(8.3e1./1.0e3);
    t815 = t753+t813+t814-t831;
    t816 = t18.*t791.*(1.1e1./1.0e2);
    t817 = t18.*t803;
    t818 = t19.*t805;
    t819 = t6.*t135.*4.5395532e-3;
    t820 = t8.*t23.*t135.*4.34580624e-2;
    t821 = t757+t817+t818+t819+t820;
    t822 = t7.*t821;
    t823 = t19.*t788.*(1.1e1./1.0e2);
    t824 = t6.*t135.*7.4634912e-2;
    t832 = t23.*t815;
    t825 = t752+t816+t822+t823+t824-t832;
    t826 = t23.*t794.*1.1812e-1;
    t828 = t69.*t800;
    t830 = t6.*t812;
    t833 = t826+t828+t830-t7.*t799.*1.1812e-1-t8.*t825;
    t834 = t8.*t812;
    t835 = t6.*t825;
    t836 = t778+t779+t834+t835-8.29000281872e-4;
    t837 = t7.*t19.*1.337379e-2;
    t838 = t723+t837;
    t843 = t7.*t18.*1.337379e-2;
    t839 = t720-t843;
    t848 = t7.*t18.*8.878859181e-4;
    t840 = t737-t848;
    t841 = t7.*t19.*8.878859181e-4;
    t842 = t740+t841;
    t844 = t19.*t838;
    t846 = t18.*t839;
    t845 = t719+t844-t846;
    t847 = t18.*t842;
    t849 = t18.*t838.*(1.1e1./1.0e2);
    t850 = t19.*t838.*(8.3e1./1.0e3);
    t865 = t18.*t839.*(8.3e1./1.0e3);
    t851 = t753+t850-t865;
    t852 = t19.*t842;
    t853 = t41.*4.780386864e-3;
    t854 = t7.*t845.*(1.1e1./1.0e2);
    t867 = t18.*t840;
    t855 = t744+t852+t853+t854-t867+3.9312916576e-4;
    t856 = t19.*t839.*(1.1e1./1.0e2);
    t857 = t19.*t840;
    t858 = t757+t847+t857;
    t859 = t7.*t858;
    t866 = t23.*t851;
    t860 = t752+t849+t856+t859-t866;
    t861 = t7.*t23.*5.133266330688e-3;
    t862 = t7.*t23.*4.34580624e-2;
    t868 = t23.*t845;
    t863 = t862-t868;
    t864 = t69.*t863;
    t869 = t19.*(t737-t848);
    t870 = t757+t847+t869;
    t871 = t7.*t870;
    t872 = t19.*(t720-t843).*(1.1e1./1.0e2);
    t873 = t752+t849-t866+t871+t872;
    t874 = t8.*t855;
    t875 = t18.^2;
    t876 = t875.*1.06974207e-2;
    t877 = t19.^2;
    t878 = t877.*1.06974207e-2;
    t879 = t876+t878+4.5395532e-3;
    t880 = t7.*t879.*(1.1e1./1.0e2);
    t881 = t875.*7.66981760273e-4;
    t882 = t877.*7.66981760273e-4;
    t883 = t880+t881+t882+5.42558408412e-4;
    t884 = t875.*8.878859181e-4;
    t885 = t877.*8.878859181e-4;
    t886 = t884+t885+4.30130092884e-4;
    t887 = t23.*t879.*1.1812e-1;
    t888 = t6.*t883;
    t889 = t8.*t23.*t886;
    t890 = t23.*t69.*t879;
    t891 = t887+t888+t889+t890;
    t892 = t8.*t883;
    t893 = t892-t6.*t23.*t886;
    t894 = t23.*t610;
    t895 = t8.*t594.*3.7397712e-2;
    t904 = t6.*t597.*3.7397712e-2;
    t905 = t7.*t644;
    t896 = t894+t895-t904-t905;
    t897 = t7.*t604.*4.5395532e-3;
    t898 = t18.*t633;
    t899 = t8.*t597.*7.4634912e-2;
    t900 = t19.*t637;
    t901 = t6.*t594.*7.4634912e-2;
    t902 = t897+t898+t899+t900+t901;
    t903 = t2.*t4.*1.04046756e-2;
    t906 = t8.*t896;
    t907 = t6.*t902;
    t909 = t3.*t5.*1.04046756e-2;
    t908 = t903+t906+t907-t909;
    t910 = t2.*t3.*1.04046756e-2;
    t911 = t4.*t5.*1.04046756e-2;
    t912 = t8.*t902;
    t913 = t910+t911+t912-t6.*t896;
    t914 = t23.*4.5395532e-3;
    t915 = t6.*t709.*6.6047e-1;
    t916 = t18.*t726;
    t917 = t19.*t722;
    t918 = t3.*t8.*t142.*6.6047e-1;
    t919 = t914+t915+t916+t917+t918;
    t920 = t23.*t733;
    t921 = t8.*t709.*3.2195e-1;
    t922 = t7.*t729;
    t926 = t3.*t6.*t142.*3.2195e-1;
    t923 = t920+t921+t922-t926+3.213061e-3;
    t924 = t8.*t919;
    t925 = t3.*t142.*1.05204;
    t927 = t924+t925-t6.*t923;
    t928 = t65.*2.2408452e-1;
    t929 = t6.*t919;
    t930 = t67.*2.2408452e-1;
    t931 = t4.*t142.*1.05204;
    t932 = t8.*t923;
    t933 = t928+t929+t930+t931+t932-1.242669648e-1;
    t934 = t7.*t794;
    t935 = t23.*t799;
    t936 = t8.*t135.*3.2195e-1;
    t937 = t934+t935+t936+3.213061e-3;
    t938 = t18.*t791;
    t939 = t19.*t788;
    t940 = t6.*t135.*6.6047e-1;
    t941 = t914+t938+t939+t940;
    t942 = t6.*t937;
    t943 = t942-t8.*t941;
    t944 = t8.*t937;
    t945 = t6.*t941;
    t946 = t928+t930+t944+t945-1.242669648e-1;
    t947 = t41.*4.34580624e-2;
    t948 = t7.*t845;
    t949 = t947+t948+3.213061e-3;
    t950 = t8.*t949;
    t951 = t18.*t838;
    t952 = t19.*(t720-t843);
    t953 = t914+t951+t952;
    t954 = t6.*t953;
    t955 = t950+t954;
    t956 = t6.*t949;
    t957 = t956-t8.*t953;
    t958 = t3.*t5.*4.0e-4;
    t959 = t7.*t665;
    t960 = t6.*t597.*3.9312916576e-4;
    t961 = t6.*t919.*1.1812e-1;
    t962 = t7.*t756;
    t963 = t8.*t709.*3.213061e-3;
    t964 = t23.*t763;
    t965 = t69.*t933;
    t966 = t8.*t923.*1.1812e-1;
    t967 = t7.*t815;
    t968 = t23.*t821;
    t969 = t69.*t946;
    t970 = t8.*t937.*1.1812e-1;
    t971 = t8.*t135.*3.213061e-3;
    t972 = t6.*t941.*1.1812e-1;
    t973 = t23.*t870;
    t974 = t8.*t949.*1.1812e-1;
    t975 = t69.*t955;
    t976 = t7.*t851;
    t977 = t6.*t953.*1.1812e-1;
    t978 = t7.*2.55503e-4;
    t979 = t7.*2.55503e-4;
    B = reshape([t5.*(t5.*2.5663597062183e-2-t2.*t3.*1.59061714944e-2-t4.*t5.*1.59061714944e-2+t5.*t142.*1.7587072e-1+t6.*t594.*4.11271808e-4+t8.*t597.*4.11271808e-4+t7.*t610.*(1.6e1./1.25e2)+t23.*t644.*(1.6e1./1.25e2)-t3.*t693+t4.*t707+t135.*t597.*1.7587072e-1+t94.*(t5.*(-1.7441664e-1)+t679+t680+t681+t682+t683-t2.*t3.*1.242669648e-1-t4.*t5.*1.242669648e-1+t5.*t142.*2.73662))+t2.*(t2.*1.2463597062183e-2+t4.*t693+t3.*t707)+1.78985264028e-2,t2.*3.0e-4+t958+t959+t960-t2.*t4.*4.0e-4-t8.*t594.*3.9312916576e-4-t23.*t656-t8.*t896.*1.1812e-1-t6.*t902.*1.1812e-1-t4.*t908.*(1.6e1./1.25e2)-t3.*t913.*(1.6e1./1.25e2)-t69.*t908-t94.*(t2.*1.188349623e-1+t4.*t908+t3.*t913),t958+t959+t960-t2.*t4.*4.0e-4-t8.*t594.*3.9312916576e-4-t23.*t656-t8.*t896.*1.1812e-1-t6.*t902.*1.1812e-1-t69.*t908,t959+t960-t8.*t594.*3.9312916576e-4-t23.*t656,-t670-t671-t672+t686+t687+t8.*t594.*5.42558408412e-4-t6.*t597.*5.42558408412e-4,t23.*t604.*2.55503e-4,-t2.*(t90.*2.89957308012e-2+t92.*2.89957308012e-2+t3.*t784+t4.*t783-1.55108751744e-2)+t5.*(t7.*t733.*(-1.6e1./1.25e2)+t23.*t729.*(1.6e1./1.25e2)+t3.*t783-t4.*t784+t94.*t734),t961+t962+t963+t964+t965+t966+t3.*t927.*(1.6e1./1.25e2)+t4.*t933.*(1.6e1./1.25e2)+t94.*(t90.*3.3248172e-1+t92.*3.3248172e-1+t3.*t927+t4.*t933-1.7441664e-1)-t3.*t6.*t142.*3.213061e-3+4.049136634878e-2,t961+t962+t963+t964+t965+t966-t3.*t6.*t142.*3.213061e-3+8.42408334878e-3,t962+t963+t964-t3.*t6.*t142.*3.213061e-3+4.6204934878e-4,-t744-t747-t750+t775,t979,t5.*(t7.*t799.*(-1.6e1./1.25e2)+t23.*t794.*(1.6e1./1.25e2)+t4.*t833+t3.*t836+t94.*t800)+t2.*(t3.*t833-t4.*t836),t967+t968+t969+t970+t971+t972-t3.*t943.*(1.6e1./1.25e2)+t4.*t946.*(1.6e1./1.25e2)-t94.*(t3.*t943-t4.*t946)+8.76204934878e-3,t967+t968+t969+t970+t971+t972+2.549136634878e-2,t967+t968+t971+4.6204934878e-4,-t744-t808-t811+t829,t979,-t5.*(t7.*t23.*5.5626319872e-3-t23.*t845.*(1.6e1./1.25e2)+t94.*t863-t3.*(t874+t6.*t873)+t4.*(t861+t864-t6.*t855-t23.*t845.*1.1812e-1+t8.*t873))-t2.*(t4.*(t874+t6.*t860)+t3.*(t861+t864-t6.*t855+t8.*t860-t23.*t845.*1.1812e-1)),t973+t974+t975+t976+t977+t4.*t955.*(1.6e1./1.25e2)-t3.*t957.*(1.6e1./1.25e2)+t94.*(t4.*t955-t3.*t957)+1.2408334878e-4,t973+t974+t975+t976+t977+1.2408334878e-4,t973+t976+1.719136634878e-2,-t744-t852+t18.*(t737-t848),t979,-t2.*(t3.*t891-t4.*t893)-t5.*(t4.*t891+t3.*t893+t23.*t879.*(1.6e1./1.25e2)+t23.*t94.*t879),-t7.*t886+t94.*(t3.*t6.*t7.*t879-t4.*t7.*t8.*t879)-t7.*t8.*t879.*1.1812e-1+t3.*t6.*t7.*t879.*(1.6e1./1.25e2)-t4.*t7.*t8.*t879.*(1.6e1./1.25e2)-t7.*t8.*t69.*t879,-t7.*t886-t7.*t8.*t879.*1.1812e-1-t7.*t8.*t69.*t879,-t7.*t886,t881+t882+1.7271875408412e-2,0.0,t2.*(t4.*t6.*t23.*2.55503e-4+t3.*t8.*t23.*2.55503e-4)-t5.*(t3.*t6.*t23.*2.55503e-4-t4.*t8.*t23.*2.55503e-4),t978,t978,t978,0.0,1.698482e-2],[6,6]);
end
